simulink model "test1"  (R2019a)
settings: Solver=VariableStepAuto  StartTime=0.0  StopTime=10.0  RelTol=1e-3
libraries: dspvision x3
settings Model: Creator=孔德岚  LastModifiedBy=孔德岚

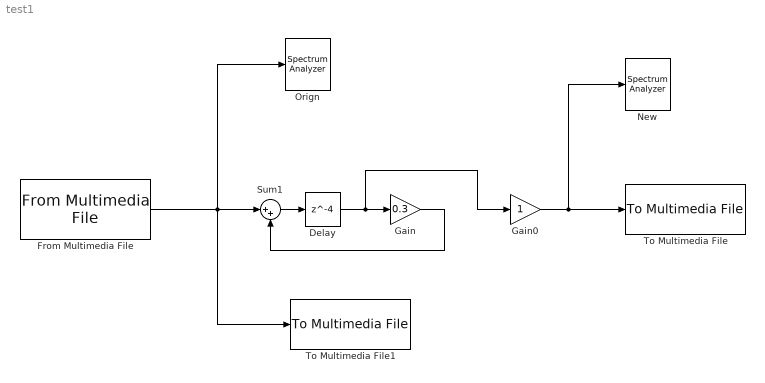
== system test1 ==
  "Delay " : Delay  DelayLength=4  InitialCondition=0
  From Multimedia File : dspvision/From Multimedia File  inputFilename=D:\Matlab\toolbox\dsp\dsp\speech_dft.mp3  readRange=[1 Inf]  loop=on  numPlays=inf  outputStreams=Audio only  videoDataType=single  audioDataType=double  inheritSampleTime=on  userDefinedSampleTime=1/30  noAudioOutput=off  isIntensityVideo=off  fourcc=RGB  colorVideoFormat=Separate color signals  outputEOF=off  dataOrg=Column-major  audioFrameSize=1024  computeAudioFrameSize=off  outSamplingMode=Sample based
      settings: SourceProductName=DSP System Toolbox  SourceProductBaseCode=DS
  "Gain " : Gain  Gain=0.3
  "Gain0 " : Gain
  "New " : SpectrumAnalyzer
  Orign : SpectrumAnalyzer
  Sum1 : Sum  Inputs=|++
  To Multimedia File : dspvision/To Multimedia File  outputFilename=output1.wav  streamSelection=Audio only  videoCompressor=None (uncompressed)  audioCompressor=None (uncompressed)  imagePorts=Separate color signals  fileType=WAV  audioDatatype=16-bit integer  fourcc=RGB  videoQuality=75  mj2000CompFactor=10
      settings: SourceProductName=DSP System Toolbox  SourceProductBaseCode=DS
  To Multimedia File1 : dspvision/To Multimedia File  outputFilename=input.wav  streamSelection=Audio only  videoCompressor=None (uncompressed)  audioCompressor=None (uncompressed)  imagePorts=Separate color signals  fileType=WAV  audioDatatype=16-bit integer  fourcc=RGB  videoQuality=75  mj2000CompFactor=10
      settings: SourceProductName=DSP System Toolbox  SourceProductBaseCode=DS
  wires:
  From Multimedia File/1 -> Sum1/1, Orign/1, To Multimedia File1/1
  "Delay "/1 -> "Gain "/1, "Gain0 "/1
  "Gain "/1 -> Sum1/2
  Sum1/1 -> "Delay "/1
  "Gain0 "/1 -> "New "/1, To Multimedia File/1
